simulink model "partage_jac"  (Simulink 7.5)
settings: Solver=ode45  StartTime=0.0  StopTime=10.0  RelTol=1e-3
settings Model: Creator=paris  LastModifiedBy=paris

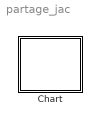
== system partage_jac ==
  Chart : Stateflow chart  TreatAsAtomicUnit=on

== stateflow chart Chart ==
  state Jugement_Adequation_Comportement
    state Conduite_Dans_Voie
    state Optimisation_Trajectoire
    state Defaut_Maitrise
    state Sortie_Voie_Legitime
    Jugement_Adequation_Comportement -> Conduite_Dans_Voie : [in(Risque_Sortie_Voie.Dans_Voie)]
    (default) -> Conduite_Dans_Voie
    Conduite_Dans_Voie -> (junction 8) : [in(Risque_Sortie_Voie.SV_Imminente) || in(Risque_Sortie_Voie.SV_Effective)]
    (junction 8) -> Optimisation_Trajectoire [order 2] : [(in(MODEL_ACTIVITE_SITUEE.franchissement_VAG.VAG_JAC_SVD) || in(MODEL_ACTIVITE_SITUEE.franchissement_VAG.Fin_Gestion_Courbe)) && in(MANOEUVRE_SV.SORTIE_VOIE.SVG)]
    (junction 8) -> Optimisation_Trajectoire [order 3] : [in(MODEL_ACTIVITE_SITUEE.franchissement_VAG.VAG_JAC_SVD) && in(MANOEUVRE_SV.SORTIE_VOIE.SVD)]
    (junction 8) -> Optimisation_Trajectoire [order 5] : [in(MODEL_ACTIVITE_SITUEE.franchissement_VAD.VAD_JAC_SVG) && in(MANOEUVRE_SV.SORTIE_VOIE.SVG) ]
    (junction 8) -> Optimisation_Trajectoire [order 4] : [in(MODEL_ACTIVITE_SITUEE.franchissement_VAD) && in(MANOEUVRE_SV.SORTIE_VOIE.SVD)]
    (junction 8) -> Defaut_Maitrise [order 6] : [ml.type_infrastructure<>62]
    (junction 8) -> Sortie_Voie_Legitime [order 1] : [ml.etat_obstacle==1]
